simulink model "pendule_inv_etu"  (R2021a)
settings: Solver=VariableStepAuto  StartTime=0.0  StopTime=10.0  RelTol=1e-3
values from neighbouring files (symbols this model uses):
  K = [10 1]    [simu_pendule_inv_capteur_etu.m]    (also in simu_pendule_inv_echant_etu.m = [30 10]; simu_pendule_inv_etu.m = [30 10])
  ue = 0    [simu_pendule_inv_capteur_etu.m]    (also in simu_pendule_inv_echant_etu.m; simu_pendule_inv_etu.m)
  x0 = [pi/20 0]'    [simu_pendule_inv_capteur_etu.m]    (also in simu_pendule_inv_echant_etu.m; simu_pendule_inv_etu.m = [pi/10 0]')
  xe = [0 0]'    [simu_pendule_inv_capteur_etu.m]    (also in simu_pendule_inv_echant_etu.m; simu_pendule_inv_etu.m)
settings Model: Creator=melyesse  LastModifiedBy=melyesse

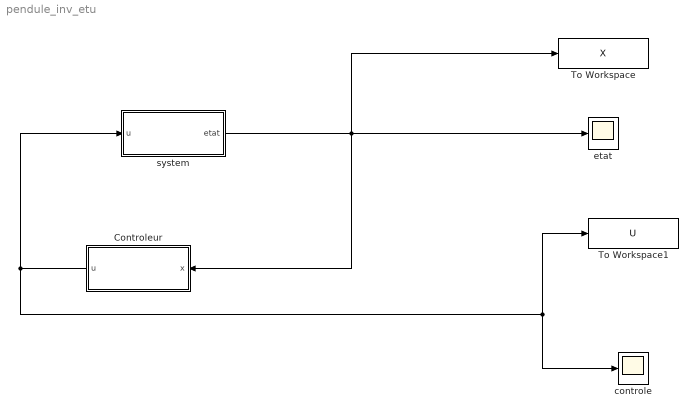
== system pendule_inv_etu ==
  Controleur : Subsystem
  To Workspace : ToWorkspace  VariableName=X  SaveFormat=Timeseries  SampleTime=-1
  To Workspace1 : ToWorkspace  VariableName=U  SaveFormat=Timeseries  SampleTime=-1
  controle : Scope
  etat : Scope
  system : Subsystem
  wires:
  Controleur/1(u) -> system/1(u), controle/1, To Workspace1/1
  system/1(etat) -> Controleur/1(x), etat/1, To Workspace/1

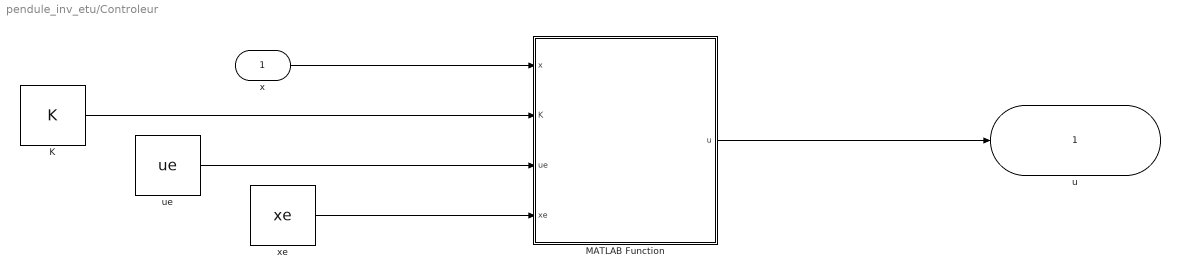
== system pendule_inv_etu/Controleur ==
  x : Inport
  K : Constant  Value=K  VectorParams1D=off
  MATLAB Function : MATLAB Function  TreatAsAtomicUnit=on
  ue : Constant  Value=ue
  xe : Constant  Value=xe
  u : Outport
  wires:
  xe/1 -> MATLAB Function/4(xe)
  ue/1 -> MATLAB Function/3(ue)
  x/1 -> MATLAB Function/1(x)
  MATLAB Function/1(u) -> u/1
  K/1 -> MATLAB Function/2(K)

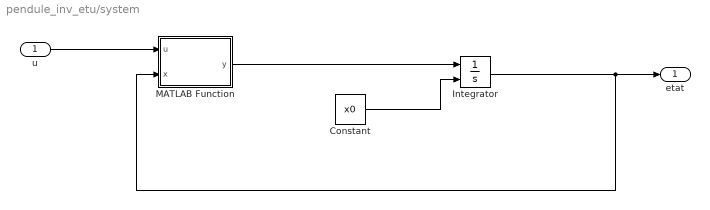
== system pendule_inv_etu/system ==
  u : Inport
  Constant : Constant  Value=x0
  Integrator : Integrator  InitialConditionSource=external
  MATLAB Function : MATLAB Function  TreatAsAtomicUnit=on
  etat : Outport
  wires:
  MATLAB Function/1(y) -> Integrator/1
  u/1 -> MATLAB Function/1(u)
  Constant/1 -> Integrator/2
  Integrator/1 -> MATLAB Function/2(x), etat/1

== matlab function pendule_inv_etu/system/MATLAB Function ==
  data: u input; y output; x input
function y = fcn(u,x)
g = 9.81;
l = 10;
y = [x(2) (((g/l)*sin(x(1)))-(cos(x(1))*u)/l)]';

== matlab function pendule_inv_etu/Controleur/MATLAB Function ==
  data: x input; u output; K input; ue input; xe input
function u = fcn(x,K,ue,xe)
u = ue + (K*(x-xe));
